simulink model "schwarchildGeodesicSolver"  (R2019b)
settings: Solver=FixedStepAuto  StartTime=0.0  StopTime=2.2  RelTol=1e-3
settings Model: Creator=jaimevrl  LastModifiedBy=jaimevrl
settings OptimizationCC: DefaultParameterBehavior=Inlined  EnhancedBackFolding=on  PassReuseOutputArgsThreshold=0  OptimizeBlockOrder=speed  DifferentSizesBufferReuse=on  OptimizationCustomize=off
settings DebuggingCC: ParameterTunabilityLossMsg=error
settings HardwareCC: TargetBitPerLong=64  TargetBitPerPointer=64  TargetBitPerSizeT=64  TargetBitPerPtrDiffT=64  TargetLongLongMode=on  TargetIntDivRoundTo=Zero  TargetEndianess=LittleEndian  TargetWordSize=64  TargetHWDeviceType=MATLAB Host  ProdEqTarget=off
settings SFSimCC: MATLABDynamicMemAlloc=off
settings RTWCC: Description=Generic Real-Time Target  GenerateReport=on  LaunchReport=on
settings CodeAppCC: ForceParamTrailComments=on  OperatorAnnotations=on

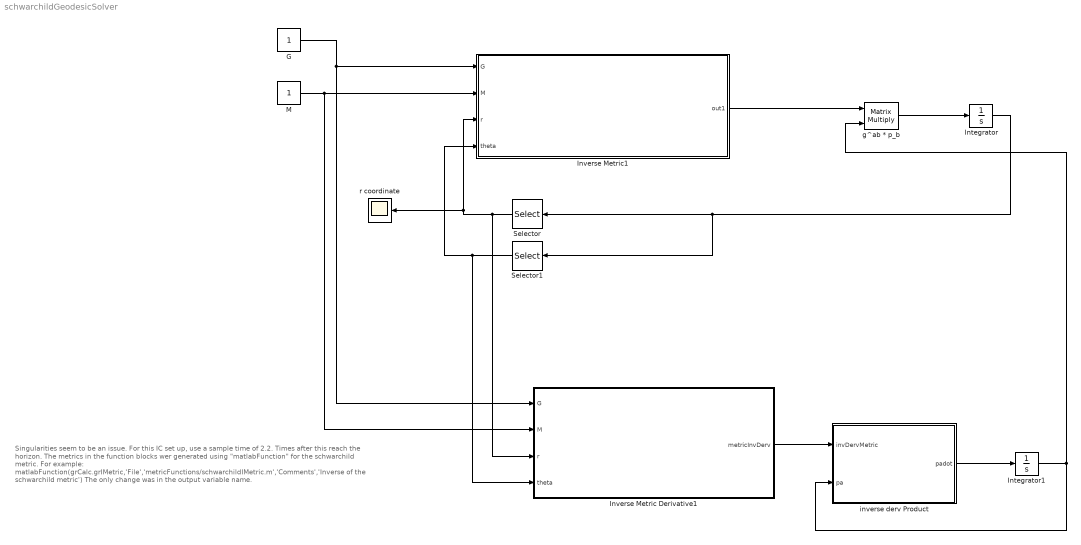
== system schwarchildGeodesicSolver ==
  note: Singularities seem to be an issue.  For this IC set up, use a sample
      | time of 2.2.  Times after this reach the horizon.
      |
      | The metrics in the function blocks
      | wer generated using "matlabFunction"
      | for the schwarchild metric. For example:
      |
      | matlabFunction(grCalc.grIMetric,'File','metricFunctions/schwarchildIMetric.m','Comments','Inverse of the schwarchild metric')
      |
      |
      | The only change was in the output variable
      | name.
  G : Constant
  Integrator : Integrator  InitialCondition=[0 3.0 3.14/2.0 0]  ContinuousStateAttributes='position'
  Integrator1 : Integrator  InitialCondition=[1.0 0 0 0]  ContinuousStateAttributes='p_a'
  Inverse Metric Derivative1 : MATLAB Function  TreatAsAtomicUnit=on
  Inverse Metric1 : MATLAB Function  TreatAsAtomicUnit=on
  M : Constant
  Selector : Selector  InputPortWidth=4  IndexOptions=Index vector (dialog)  Indices=[2]  OutputSizes=1
  Selector1 : Selector  InputPortWidth=4  IndexOptions=Index vector (dialog)  Indices=[3]  OutputSizes=1
  g^ab * p_b : Product  Multiplication=Matrix(*)
  inverse derv Product : MATLAB Function  TreatAsAtomicUnit=on
  r coordinate : Scope
  wires:
  G/1 -> Inverse Metric Derivative1/1(G), Inverse Metric1/1(G)
  M/1 -> Inverse Metric Derivative1/2(M), Inverse Metric1/2(M)
  Inverse Metric1/1(out1) -> g^ab * p_b/1
  g^ab * p_b/1 -> Integrator/1
  Integrator/1 -> Selector1/1, Selector/1
  Selector1/1 -> Inverse Metric Derivative1/4(theta), Inverse Metric1/4(theta)
  Integrator1/1 -> g^ab * p_b/2, inverse derv Product/2(pa)
  inverse derv Product/1(padot) -> Integrator1/1
  Inverse Metric Derivative1/1(metricInvDerv) -> inverse derv Product/1(invDervMetric)
  Selector/1 -> Inverse Metric Derivative1/3(r), Inverse Metric1/3(r), r coordinate/1

== matlab function schwarchildGeodesicSolver/Inverse Metric1 ==
  data: G input; out1 output; M input; r input; theta input
function out1 = schwarchildIMetric(G,M,r,theta)
%SCHWARCHILDIMETRIC
%    OUT1 = SCHWARCHILDIMETRIC(G,M,R,THETA)

%    This function was generated by the Symbolic Math Toolbox version 8.4.
%    11-Mar-2020 23:24:46

%Inverse of the schwarchild metric
t2 = 1.0./r.^2;
t3 = G.*M.*2.0;
t4 = -t3;
t5 = r+t4;
out1 = reshape([-r./t5,0.0,0.0,0.0,0.0,t5./r,0.0,0.0,0.0,0.0,t2,0.0,0.0,0.0,0.0,t2.*1.0./sin(theta).^2],[4,4]);

== matlab function schwarchildGeodesicSolver/inverse derv Product ==
  data: invDervMetric input; padot output; pa input
function padot = inverseDervProduct(invDervMetric,pa)
% pdot_a = p_b * p_c * dg^{bc}/dx^a
%   Detailed explanation goes here
dim = length(pa);
padot = zeros(dim,1);
for a = 1 : dim
   padot(a) = -0.5 * dot(pa, invDervMetric(:,:,a) * pa); 
end
end

== matlab function schwarchildGeodesicSolver/Inverse Metric Derivative1 ==
  data: G input; metricInvDerv output; M input; r input; theta input
function metricInvDerv = schwarchildIMetricDerv(G,M,r,theta)
%SCHWARCHILDIMETRICDERV
%    OUT1 = SCHWARCHILDIMETRICDERV(G,M,R,THETA)

%    This function was generated by the Symbolic Math Toolbox version 8.4.
%    11-Mar-2020 22:09:38

%Inverse derivative of the schwarchild metric
t2 = sin(theta);
t3 = 1.0./r.^3;
t4 = G.*M.*2.0;
t5 = -t4;
t6 = r+t5;
metricInvDerv = reshape([0.0,0.0,0.0,0.0,0.0,0.0,0.0,0.0,0.0,0.0,0.0,0.0,0.0,0.0,0.0,0.0,t4.*1.0./t6.^2,0.0,0.0,0.0,0.0,1.0./r.^4.*t4.*t6.^2.*1.0./(t4./r-1.0).^2,0.0,0.0,0.0,0.0,t3.*-2.0,0.0,0.0,0.0,0.0,1.0./t2.^2.*t3.*-2.0,0.0,0.0,0.0,0.0,0.0,0.0,0.0,0.0,0.0,0.0,0.0,0.0,0.0,0.0,0.0,1.0./r.^2.*1.0./t2.^3.*cos(theta).*-2.0,0.0,0.0,0.0,0.0,0.0,0.0,0.0,0.0,0.0,0.0,0.0,0.0,0.0,0.0,0.0,0.0],[4,4,4]);
